simulink model "Follower_V2V_Solyom2013"  (R2014b)
settings: Solver=ode3  SolverMode=SingleTasking  StartTime=0.0  StopTime=10.0  FixedStep=sampleTimes.main  RelTol=1e-3
model workspace (MAT data in the model file):
  spacing = 0
  vehicle = 0
undefined symbols (not defined in the file or in its folder): delays
libraries: simulink x12
settings Model: ParameterArgumentNames=vehicle,spacing  Creator=uos  LastModifiedBy=uos

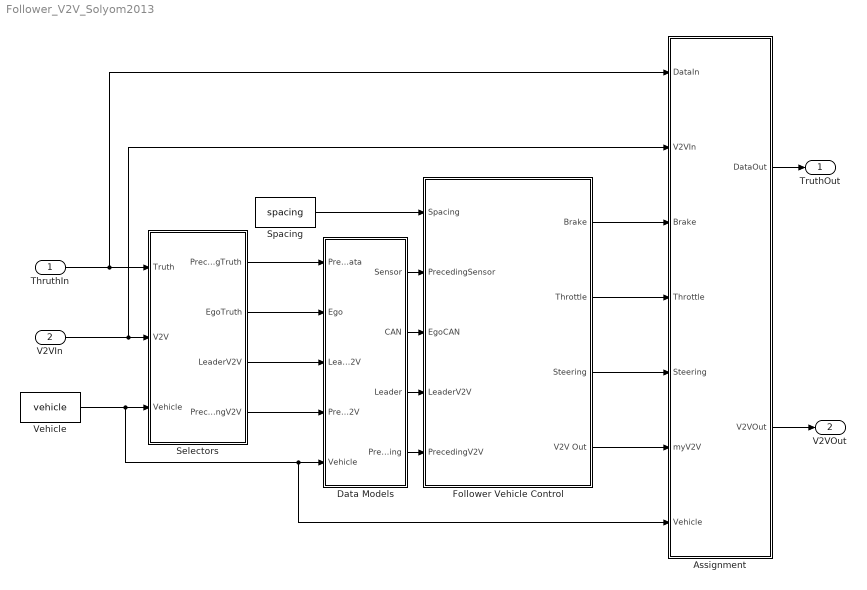
== system Follower_V2V_Solyom2013 ==
  ThruthIn : Inport  OutDataTypeStr=Bus: VehicleBus  PortDimensions=10  BusOutputAsStruct=on
  V2VIn : Inport  Port=2  OutDataTypeStr=Bus: V2VBus  PortDimensions=10  SampleTime=0  BusOutputAsStruct=on
  Assignment : Subsystem
  Data Models : Subsystem
  Follower Vehicle Control : Subsystem
  Selectors : Subsystem
  Spacing : Constant  Value=spacing
  Vehicle : Constant  Value=vehicle
  TruthOut : Outport  OutDataTypeStr=Bus: VehicleBus  PortDimensions=10  BusOutputAsStruct=on
  V2VOut : Outport  Port=2  OutDataTypeStr=Bus: V2VBus  PortDimensions=10  BusOutputAsStruct=on
  wires:
  ThruthIn/1 -> Assignment/1(DataIn), Selectors/1(Truth)
  Assignment/1(DataOut) -> TruthOut/1
  Spacing/1 -> Follower Vehicle Control/1(Spacing)
  Vehicle/1 -> Assignment/7(Vehicle), Data Models/5(Vehicle), Selectors/3(Vehicle)
  Follower Vehicle Control/1(Brake) -> Assignment/3(Brake)
  Follower Vehicle Control/2(Throttle) -> Assignment/4(Throttle)
  Follower Vehicle Control/3(Steering) -> Assignment/5(Steering)
  V2VIn/1 -> Assignment/2(V2VIn), Selectors/2(V2V)
  Assignment/2(V2VOut) -> V2VOut/1
  Follower Vehicle Control/4(V2V Out) -> Assignment/6(myV2V)
  Selectors/1(PrecedingTruth) -> Data Models/1(PrecedingData)
  Selectors/2(EgoTruth) -> Data Models/2(Ego)
  Selectors/3(LeaderV2V) -> Data Models/3(LeaderV2V)
  Selectors/4(PrecedingV2V) -> Data Models/4(PrecedingV2V)
  Data Models/1(Sensor) -> Follower Vehicle Control/2(PrecedingSensor)
  Data Models/2(CAN) -> Follower Vehicle Control/3(EgoCAN)
  Data Models/3(Leader) -> Follower Vehicle Control/4(LeaderV2V)
  Data Models/4(Preceding) -> Follower Vehicle Control/5(PrecedingV2V)

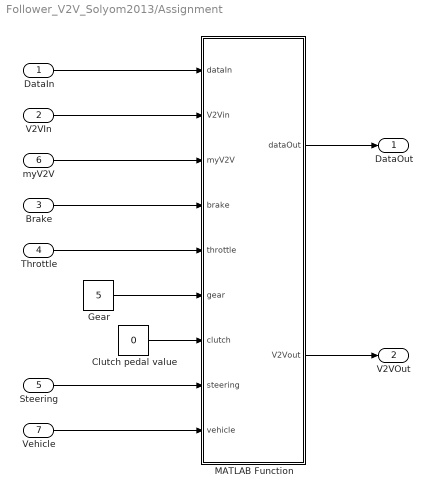
== system Follower_V2V_Solyom2013/Assignment ==
  DataIn : Inport
  V2VIn : Inport  Port=2
  Brake : Inport  Port=3
  Throttle : Inport  Port=4
  Steering : Inport  Port=5
  myV2V : Inport  Port=6
  Vehicle : Inport  Port=7
  Clutch pedal value : Constant  Value=0
  Gear : Constant  Value=5  OutDataTypeStr=int32
  MATLAB Function : MATLAB Function  TreatAsAtomicUnit=on
  DataOut : Outport
  V2VOut : Outport  Port=2
  wires:
  Vehicle/1 -> MATLAB Function/9(vehicle)
  DataIn/1 -> MATLAB Function/1(dataIn)
  Brake/1 -> MATLAB Function/4(brake)
  MATLAB Function/1(dataOut) -> DataOut/1
  Throttle/1 -> MATLAB Function/5(throttle)
  Steering/1 -> MATLAB Function/8(steering)
  V2VIn/1 -> MATLAB Function/2(V2Vin)
  myV2V/1 -> MATLAB Function/3(myV2V)
  MATLAB Function/2(V2Vout) -> V2VOut/1
  Gear/1 -> MATLAB Function/6(gear)
  Clutch pedal value/1 -> MATLAB Function/7(clutch)

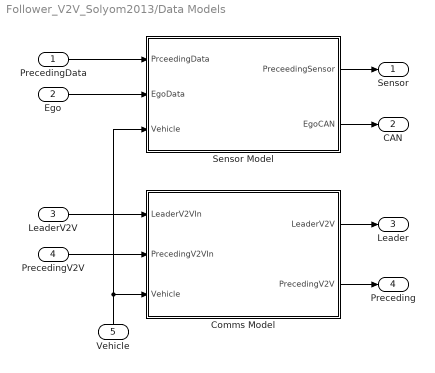
== system Follower_V2V_Solyom2013/Data Models ==
  PrecedingData : Inport
  Ego : Inport  Port=2
  LeaderV2V : Inport  Port=3
  PrecedingV2V : Inport  Port=4
  Vehicle : Inport  Port=5
  Comms Model : Subsystem
  Sensor Model : Subsystem
  Sensor : Outport
  CAN : Outport  Port=2
  Leader : Outport  Port=3
  Preceding : Outport  Port=4
  wires:
  Sensor Model/2(EgoCAN) -> CAN/1
  Sensor Model/1(PreceedingSensor) -> Sensor/1
  PrecedingData/1 -> Sensor Model/1(PrceedingData)
  Ego/1 -> Sensor Model/2(EgoData)
  LeaderV2V/1 -> Comms Model/1(LeaderV2VIn)
  PrecedingV2V/1 -> Comms Model/2(PrecedingV2VIn)
  Comms Model/1(LeaderV2V) -> Leader/1
  Comms Model/2(PrecedingV2V) -> Preceding/1
  Vehicle/1 -> Sensor Model/3(Vehicle), Comms Model/3(Vehicle)

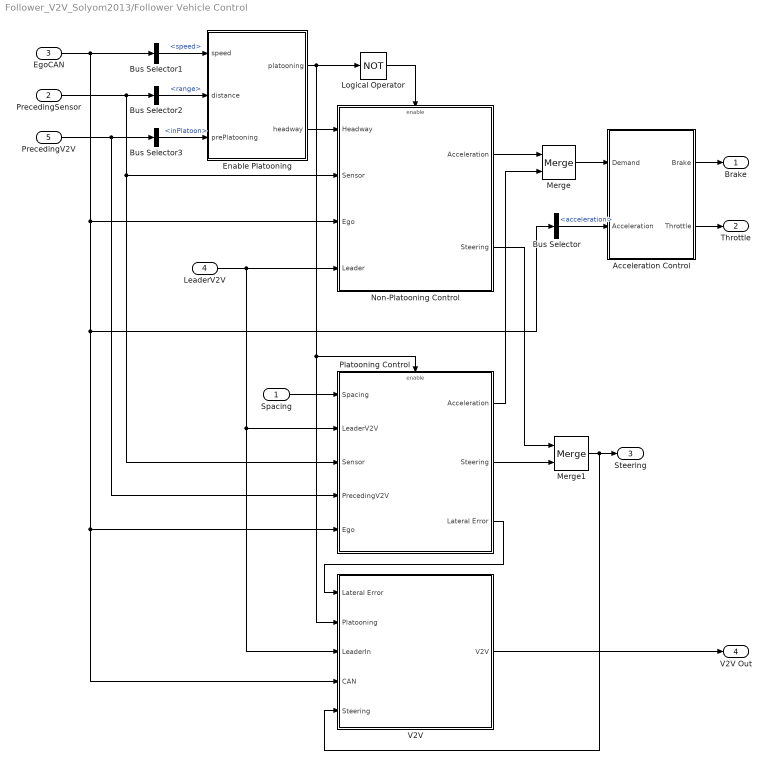
== system Follower_V2V_Solyom2013/Follower Vehicle Control ==
  Spacing : Inport
  PrecedingSensor : Inport  Port=2
  EgoCAN : Inport  Port=3
  LeaderV2V : Inport  Port=4
  PrecedingV2V : Inport  Port=5
  Acceleration Control : Subsystem
  Bus Selector : BusSelector  OutputSignals=acceleration
  Bus Selector1 : BusSelector  OutputSignals=speed
  Bus Selector2 : BusSelector  OutputSignals=range
  Bus Selector3 : BusSelector  OutputSignals=inPlatoon
  Enable Platooning : Stateflow chart  TreatAsAtomicUnit=on
  Logical Operator : Logic  Operator=NOT  AllPortsSameDT=off  OutDataTypeStr=boolean
  Merge : Merge
  Merge1 : Merge
  Non-Platooning Control : Subsystem
  Platooning Control : Subsystem
  V2V : Subsystem
  Brake : Outport
  Throttle : Outport  Port=2
  Steering : Outport  Port=3
  V2V Out : Outport  Port=4
  wires:
  Bus Selector/1 -> Acceleration Control/2(Acceleration)  "<acceleration>"
  Acceleration Control/1(Brake) -> Brake/1
  Acceleration Control/2(Throttle) -> Throttle/1
  Merge1/1 -> Steering/1, V2V/5(Steering)
  Spacing/1 -> Platooning Control/1(Spacing)
  LeaderV2V/1 -> Non-Platooning Control/4(Leader), V2V/3(LeaderIn), Platooning Control/2(LeaderV2V)
  PrecedingSensor/1 -> Platooning Control/3(Sensor), Non-Platooning Control/2(Sensor), Bus Selector2/1
  Merge/1 -> Acceleration Control/1(Demand)
  Platooning Control/1(Acceleration) -> Merge/2
  Non-Platooning Control/1(Acceleration) -> Merge/1
  Platooning Control/2(Steering) -> Merge1/2
  Enable Platooning/1(platooning) -> V2V/2(Platooning), Platooning Control/Enable, Logical Operator/1
  Logical Operator/1 -> Non-Platooning Control/Enable
  Bus Selector1/1 -> Enable Platooning/1(speed)  "<speed>"
  Bus Selector2/1 -> Enable Platooning/2(distance)  "<range>"
  EgoCAN/1 -> Bus Selector1/1, Non-Platooning Control/3(Ego), V2V/4(CAN), Platooning Control/5(Ego), Bus Selector/1
  V2V/1(V2V) -> V2V Out/1
  Enable Platooning/2(headway) -> Non-Platooning Control/1(Headway)
  PrecedingV2V/1 -> Bus Selector3/1, Platooning Control/4(PrecedingV2V)
  Platooning Control/3(Lateral Error) -> V2V/1(Lateral Error)
  Bus Selector3/1 -> Enable Platooning/3(prePlatooning)  "<inPlatoon>"
  Non-Platooning Control/2(Steering) -> Merge1/1

== system Follower_V2V_Solyom2013/Selectors ==
  Truth : Inport
  V2V : Inport  Port=2
  Vehicle : Inport  Port=3
  MATLAB Function : MATLAB Function  TreatAsAtomicUnit=on
  PrecedingTruth : Outport
  EgoTruth : Outport  Port=2
  LeaderV2V : Outport  Port=3
  PrecedingV2V : Outport  Port=4
  wires:
  Truth/1 -> MATLAB Function/1(data)
  Vehicle/1 -> MATLAB Function/3(vehicle)
  MATLAB Function/2(egoTruth) -> EgoTruth/1
  V2V/1 -> MATLAB Function/2(V2V)
  MATLAB Function/3(leaderV2V) -> LeaderV2V/1
  MATLAB Function/4(precedingV2V) -> PrecedingV2V/1
  MATLAB Function/1(precedingTruth) -> PrecedingTruth/1

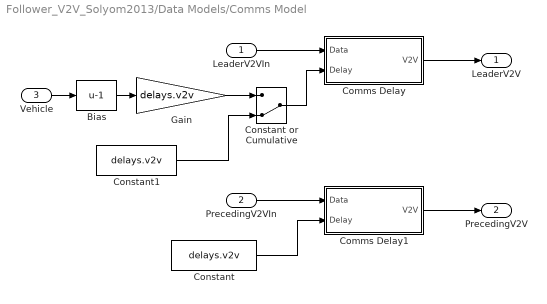
== system Follower_V2V_Solyom2013/Data Models/Comms Model ==
  LeaderV2VIn : Inport
  PrecedingV2VIn : Inport  Port=2
  Vehicle : Inport  Port=3
  Bias : Bias  Bias=-1
  Comms Delay : Subsystem
  Comms Delay1 : Subsystem
  Constant : Constant  Value=delays.v2v
  Constant or Cumulative : ManualSwitch  CurrentSetting=0
  Constant1 : Constant  Value=delays.v2v
  Gain : Gain  Gain=delays.v2v
  LeaderV2V : Outport
  PrecedingV2V : Outport  Port=2
  wires:
  LeaderV2VIn/1 -> Comms Delay/1(Data)
  Comms Delay/1(V2V) -> LeaderV2V/1
  PrecedingV2VIn/1 -> Comms Delay1/1(Data)
  Comms Delay1/1(V2V) -> PrecedingV2V/1
  Constant/1 -> Comms Delay1/2(Delay)
  Constant or Cumulative/1 -> Comms Delay/2(Delay)
  Constant1/1 -> Constant or Cumulative/2
  Vehicle/1 -> Bias/1
  Bias/1 -> Gain/1
  Gain/1 -> Constant or Cumulative/1

== system Follower_V2V_Solyom2013/Data Models/Sensor Model ==
  PrceedingData : Inport
  EgoData : Inport  Port=2
  Vehicle : Inport  Port=3
  CAN Model : Subsystem
  Radar Model : Subsystem
  PreceedingSensor : Outport
  EgoCAN : Outport  Port=2
  wires:
  EgoData/1 -> CAN Model/1(Data), Radar Model/2(Ego)
  Radar Model/1(Radar Data) -> PreceedingSensor/1
  CAN Model/1(CAN) -> EgoCAN/1
  PrceedingData/1 -> Radar Model/1(Target)
  Vehicle/1 -> CAN Model/2(Vehicle)

== system Follower_V2V_Solyom2013/Follower Vehicle Control/Acceleration Control ==
  Demand : Inport
  Acceleration : Inport  Port=2
  Brake Control : Subsystem
  Compare To Constant : simulink/Logic and Bit Operations/Compare To Constant  relop=>=  const=-0.1  OutDataTypeStr=boolean
  Logical Operator : Logic  Operator=NOT  AllPortsSameDT=off  OutDataTypeStr=boolean
  Sum1 : Sum  Inputs=+-|
  Throttle Control : Subsystem
  Brake : Outport
  Throttle : Outport  Port=2
  wires:
  Acceleration/1 -> Throttle Control/2(Acceleration), Sum1/2
  Demand/1 -> Throttle Control/1(Demand), Compare To Constant/1, Sum1/1
  Sum1/1 -> Brake Control/1(Error)
  Brake Control/1(Brake) -> Brake/1
  Throttle Control/1(Throttle) -> Throttle/1
  Compare To Constant/1 -> Throttle Control/Enable, Logical Operator/1
  Logical Operator/1 -> Brake Control/Enable

== system Follower_V2V_Solyom2013/Follower Vehicle Control/Non-Platooning Control ==
  Headway : Inport
  Sensor : Inport  Port=2
  Ego : Inport  Port=3
  Leader : Inport  Port=4
  Enable : EnablePort
  Speed Control : Subsystem
  Steering Control : Subsystem
  Steering Control1 : Subsystem
  Acceleration : Outport
  Steering : Outport  Port=2
  wires:
  Steering Control1/1(Target Curvature) -> Steering Control/2(Target Curvature)
  Ego/1 -> Steering Control/1(Ego), Speed Control/2(Ego)
  Sensor/1 -> Steering Control1/1(Sensor), Speed Control/3(Leader)
  Headway/1 -> Speed Control/1(Headway)
  Speed Control/1(Acceleration Demand) -> Acceleration/1
  Leader/1 -> Steering Control1/2(Leader)
  Steering Control/1(Steering) -> Steering/1

== system Follower_V2V_Solyom2013/Follower Vehicle Control/Platooning Control ==
  Spacing : Inport
  LeaderV2V : Inport  Port=2
  Sensor : Inport  Port=3
  PrecedingV2V : Inport  Port=4
  Ego : Inport  Port=5
  Enable : EnablePort
  Speed Control : Subsystem
  Steering Control : Subsystem
  Acceleration : Outport
  Steering : Outport  Port=2
  Lateral Error : Outport  Port=3
  wires:
  Speed Control/1(Acceleration Demand) -> Acceleration/1
  Spacing/1 -> Speed Control/1(Spacing)
  Sensor/1 -> Steering Control/2(Sensor), Speed Control/3(PreceedingSensor)
  LeaderV2V/1 -> Speed Control/2(LeaderV2V)
  PrecedingV2V/1 -> Steering Control/1(Preceeding), Speed Control/4(PreceedingV2V)
  Ego/1 -> Steering Control/3(Ego), Speed Control/5(Ego)
  Steering Control/1(Steering) -> Steering/1
  Steering Control/2(lateralError1) -> Lateral Error/1

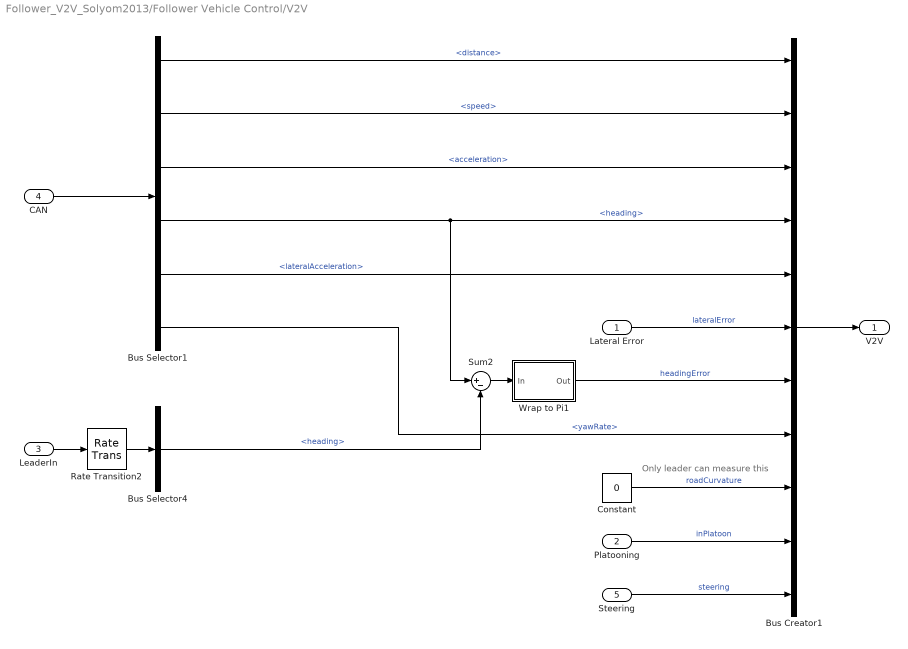
== system Follower_V2V_Solyom2013/Follower Vehicle Control/V2V ==
  note: Only leader can measure this
  Lateral Error : Inport
  Platooning : Inport  Port=2
  LeaderIn : Inport  Port=3
  CAN : Inport  Port=4
  Steering : Inport  Port=5
  Bus Creator1 : BusCreator  Inputs=11  OutDataTypeStr=Bus: V2VBus  NonVirtualBus=on
  Bus Selector1 : BusSelector  OutputSignals=distance,speed,acceleration,heading,lateralAcceleration,yawRate
  Bus Selector4 : BusSelector  OutputSignals=heading
  Constant : Constant  Value=0
  Rate Transition2 : RateTransition  OutPortSampleTime=sampleTimes.control
  Sum2 : Sum  Inputs=|+-
  Wrap to Pi1 : Subsystem
  V2V : Outport
  wires:
  CAN/1 -> Bus Selector1/1
  Bus Selector1/6 -> Bus Creator1/8  "<yawRate>"
  Constant/1 -> Bus Creator1/9  "roadCurvature"
  Bus Selector1/3 -> Bus Creator1/3  "<acceleration>"
  Bus Selector1/1 -> Bus Creator1/1  "<distance>"
  Bus Selector1/2 -> Bus Creator1/2  "<speed>"
  Bus Selector1/5 -> Bus Creator1/5  "<lateralAcceleration>"
  Bus Creator1/1 -> V2V/1
  Bus Selector1/4 -> Bus Creator1/4, Sum2/1  "<heading>"
  Sum2/1 -> Wrap to Pi1/1(In)
  LeaderIn/1 -> Rate Transition2/1
  Rate Transition2/1 -> Bus Selector4/1
  Bus Selector4/1 -> Sum2/2  "<heading>"
  Wrap to Pi1/1(Out) -> Bus Creator1/7  "headingError"
  Lateral Error/1 -> Bus Creator1/6  "lateralError"
  Platooning/1 -> Bus Creator1/10  "inPlatoon"
  Steering/1 -> Bus Creator1/11  "steering"

== system Follower_V2V_Solyom2013/Data Models/Comms Model/Comms Delay ==
  Data : Inport
  Delay : Inport  Port=2
  Display : Display
  Rate Transition1 : RateTransition  OutPortSampleTime=sampleTimes.v2v
  Rate Transition2 : RateTransition  OutPortSampleTime=sampleTimes.main
  Variable Integer Delay : Delay  DelayLengthSource=Input port
      settings: InputPortMap=u0,p1
  Weighted Sample Time Math : SampleTimeMath  TsampMathOp=/
  V2V : Outport
  wires:
  Rate Transition1/1 -> V2V/1
  Data/1 -> Rate Transition2/1
  Rate Transition2/1 -> Variable Integer Delay/1
  Delay/1 -> Weighted Sample Time Math/1
  Weighted Sample Time Math/1 -> Display/1, Variable Integer Delay/2
  Variable Integer Delay/1 -> Rate Transition1/1

== system Follower_V2V_Solyom2013/Data Models/Comms Model/Comms Delay1 ==
  Data : Inport
  Delay : Inport  Port=2
  Rate Transition1 : RateTransition  OutPortSampleTime=sampleTimes.v2v
  Rate Transition2 : RateTransition  OutPortSampleTime=sampleTimes.main
  Variable Integer Delay : Delay  DelayLengthSource=Input port
      settings: InputPortMap=u0,p1
  Weighted Sample Time Math : SampleTimeMath  TsampMathOp=/
  V2V : Outport
  wires:
  Variable Integer Delay/1 -> Rate Transition1/1
  Weighted Sample Time Math/1 -> Variable Integer Delay/2
  Delay/1 -> Weighted Sample Time Math/1
  Rate Transition2/1 -> Variable Integer Delay/1
  Data/1 -> Rate Transition2/1
  Rate Transition1/1 -> V2V/1

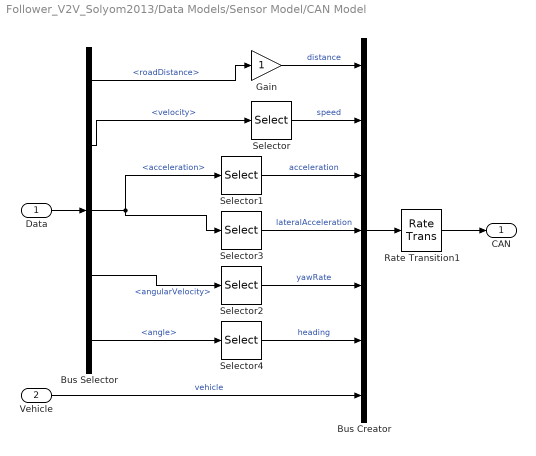
== system Follower_V2V_Solyom2013/Data Models/Sensor Model/CAN Model ==
  Data : Inport
  Vehicle : Inport  Port=2
  Bus Creator : BusCreator  Inputs=7
  Bus Selector : BusSelector  OutputSignals=data.roadDistance,data.velocity,data.acceleration,data.angularVelocity,data.angle
  Gain : Gain
  Rate Transition1 : RateTransition  OutPortSampleTime=sampleTimes.main
  Selector : Selector  InputPortWidth=3
  Selector1 : Selector  InputPortWidth=3
  Selector2 : Selector  InputPortWidth=3  Indices=3
  Selector3 : Selector  InputPortWidth=3  Indices=2
  Selector4 : Selector  InputPortWidth=3  Indices=3
  CAN : Outport
  wires:
  Rate Transition1/1 -> CAN/1
  Bus Creator/1 -> Rate Transition1/1
  Selector1/1 -> Bus Creator/3  "acceleration"
  Bus Selector/3 -> Selector1/1, Selector3/1  "<acceleration>"
  Selector/1 -> Bus Creator/2  "speed"
  Bus Selector/2 -> Selector/1  "<velocity>"
  Data/1 -> Bus Selector/1
  Bus Selector/4 -> Selector2/1  "<angularVelocity>"
  Selector2/1 -> Bus Creator/5  "yawRate"
  Selector3/1 -> Bus Creator/4  "lateralAcceleration"
  Bus Selector/5 -> Selector4/1  "<angle>"
  Selector4/1 -> Bus Creator/6  "heading"
  Bus Selector/1 -> Gain/1  "<roadDistance>"
  Gain/1 -> Bus Creator/1  "distance"
  Vehicle/1 -> Bus Creator/7  "vehicle"

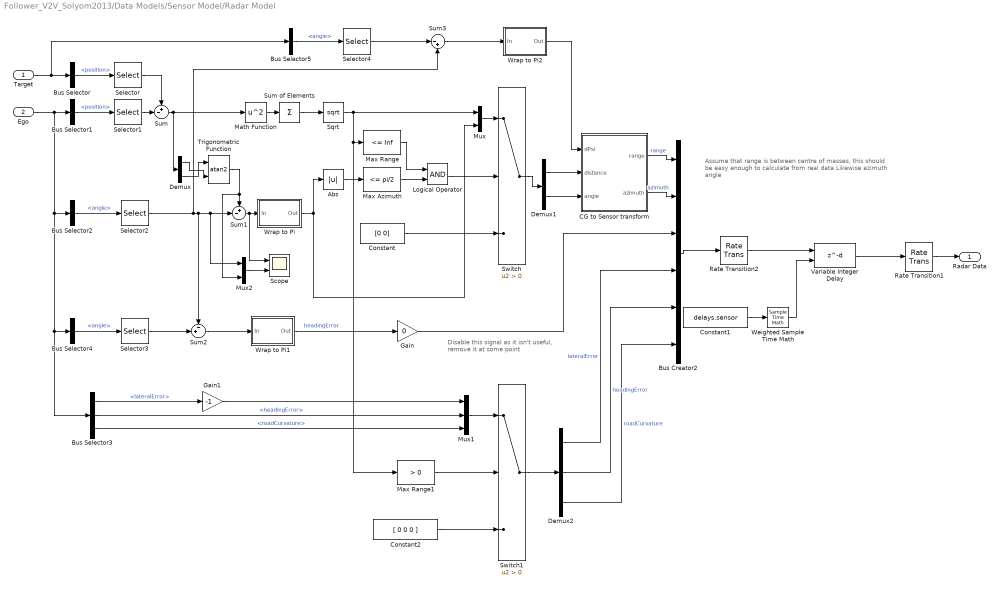
== system Follower_V2V_Solyom2013/Data Models/Sensor Model/Radar Model ==
  note: Assume that range is between centre of masses,
      | this should be easy enough to calculate from real data
      | Likewise azimuth angle
  note: Disable this signal as it isn't useful,
      | remove it at some point
  Target : Inport
  Ego : Inport  Port=2
  Abs : Abs
  Bus Creator2 : BusCreator  Inputs=6
  Bus Selector : BusSelector  OutputSignals=data.position
  Bus Selector1 : BusSelector  OutputSignals=data.position
  Bus Selector2 : BusSelector  OutputSignals=data.angle
  Bus Selector3 : BusSelector  OutputSignals=data.lateralError,data.headingError,data.roadCurvature
  Bus Selector4 : BusSelector  OutputSignals=data.angle
  Bus Selector5 : BusSelector  OutputSignals=data.angle
  CG to Sensor transform : Subsystem
  Constant : Constant  Value=[0 0]
  Constant1 : Constant  Value=delays.sensor
  Constant2 : Constant  Value=[ 0 0 0 ]
  Demux : Demux  Outputs=2
  Demux1 : Demux  Outputs=2
  Demux2 : Demux  Outputs=3
  Gain : Gain  Gain=0
  Gain1 : Gain  Gain=-1
  Logical Operator : Logic  AllPortsSameDT=off  OutDataTypeStr=boolean
  Math Function : Math  Operator=square  SaturateOnIntegerOverflow=on
  Max Azimuth : simulink/Logic and Bit Operations/Compare To Constant  relop=<=  const=pi/2  OutDataTypeStr=boolean
  Max Range : simulink/Logic and Bit Operations/Compare To Constant  relop=<=  const=Inf  OutDataTypeStr=boolean
  Max Range1 : simulink/Logic and Bit Operations/Compare To Constant  relop=>  const=0  OutDataTypeStr=boolean
  Mux : Mux  Inputs=2
  Mux1 : Mux  Inputs=3
  Mux2 : Mux  Inputs=2
  Rate Transition1 : RateTransition  OutPortSampleTime=sampleTimes.sensor
  Rate Transition2 : RateTransition  OutPortSampleTime=sampleTimes.main
  Scope : Scope  NumInputPorts=2
      settings: YMin=-5~-5  YMax=5~5  SaveName=ScopeData11
  Selector : Selector  InputPortWidth=3  Indices=[1 2]
  Selector1 : Selector  InputPortWidth=3  Indices=[1 2]
  Selector2 : Selector  InputPortWidth=3  Indices=3
  Selector3 : Selector  InputPortWidth=3  Indices=3
  Selector4 : Selector  InputPortWidth=3  Indices=3
  Sqrt : Sqrt  SaturateOnIntegerOverflow=on
  Sum : Sum  Inputs=+-|
  Sum of Elements : Sum  Inputs=+
  Sum1 : Sum  Inputs=+-|
  Sum2 : Sum  Inputs=-+|
  Sum3 : Sum  Inputs=|-+
  Switch : Switch  Criteria=u2 > Threshold
  Switch1 : Switch  Criteria=u2 > Threshold
  Trigonometric Function : Trigonometry  Operator=atan2
  Variable Integer Delay : Delay  DelayLengthSource=Input port
      settings: InputPortMap=u0,p1
  Weighted Sample Time Math : SampleTimeMath  TsampMathOp=/
  Wrap to Pi : Subsystem
  Wrap to Pi1 : Subsystem
  Wrap to Pi2 : Subsystem
  Radar Data : Outport
  wires:
  Selector1/1 -> Sum/2
  Selector/1 -> Sum/1
  Bus Selector/1 -> Selector/1  "<position>"
  Bus Selector1/1 -> Selector1/1  "<position>"
  Bus Selector2/1 -> Selector2/1  "<angle>"
  Sum/1 -> Math Function/1, Demux/1
  Selector2/1 -> Sum2/1, Mux2/1, Sum1/2, Sum3/2
  Trigonometric Function/1 -> Mux2/2, Sum1/1
  Sum1/1 -> Scope/1, Wrap to Pi/1(In)
  Math Function/1 -> Sum of Elements/1
  Sum of Elements/1 -> Sqrt/1
  Constant/1 -> Switch/3
  Logical Operator/1 -> Switch/2
  Max Range/1 -> Logical Operator/1
  Abs/1 -> Max Azimuth/1
  Max Azimuth/1 -> Logical Operator/2
  Demux/1 -> Trigonometric Function/2
  Demux/2 -> Trigonometric Function/1
  Wrap to Pi/1(Out) -> Mux/2, Abs/1
  Bus Creator2/1 -> Rate Transition2/1
  Rate Transition1/1 -> Radar Data/1
  Rate Transition2/1 -> Variable Integer Delay/1
  Variable Integer Delay/1 -> Rate Transition1/1
  Constant1/1 -> Weighted Sample Time Math/1
  Weighted Sample Time Math/1 -> Variable Integer Delay/2
  Bus Selector4/1 -> Selector3/1  "<angle>"
  Selector3/1 -> Sum2/2
  Sum2/1 -> Wrap to Pi1/1(In)
  Demux1/2 -> CG to Sensor transform/3(angle)
  Mux/1 -> Switch/1
  Sqrt/1 -> Mux/1, Max Range1/1, Max Range/1
  Switch/1 -> Demux1/1
  Wrap to Pi1/1(Out) -> Gain/1  "headingError"
  Gain/1 -> Bus Creator2/3
  Ego/1 -> Bus Selector2/1, Bus Selector3/1, Bus Selector4/1, Bus Selector1/1
  Mux1/1 -> Switch1/1
  Bus Selector3/1 -> Gain1/1  "<lateralError>"
  Bus Selector3/2 -> Mux1/2  "<headingError>"
  Max Range1/1 -> Switch1/2
  Constant2/1 -> Switch1/3
  Switch1/1 -> Demux2/1
  Demux2/1 -> Bus Creator2/4  "lateralError"
  Demux2/2 -> Bus Creator2/5  "headingError"
  Bus Selector3/3 -> Mux1/3  "<roadCurvature>"
  Demux2/3 -> Bus Creator2/6  "roadCurvature"
  Mux2/1 -> Scope/2
  Gain1/1 -> Mux1/1
  Bus Selector5/1 -> Selector4/1  "<angle>"
  Target/1 -> Bus Selector5/1, Bus Selector/1
  Selector4/1 -> Sum3/1
  Sum3/1 -> Wrap to Pi2/1(In)
  Wrap to Pi2/1(Out) -> CG to Sensor transform/1(dPsi)
  CG to Sensor transform/1(range) -> Bus Creator2/1  "range"
  CG to Sensor transform/2(azimuth) -> Bus Creator2/2  "azimuth"
  Demux1/1 -> CG to Sensor transform/2(distance)

== system Follower_V2V_Solyom2013/Follower Vehicle Control/Acceleration Control/Brake Control ==
  Error : Inport
  Enable : EnablePort  StatesWhenEnabling=reset
  Discrete-Time Integrator : DiscreteIntegrator  InitialConditionSetting=State (most efficient)  SampleTime=-1  LimitOutput=on  UpperSaturationLimit=1  LowerSaturationLimit=-1
  Gain2 : Gain  Gain=0.005
  Gain3 : Gain
  Saturation1 : Saturate  UpperLimit=1  LowerLimit=0
  Sum2 : Sum  Inputs=++|
  Unary Minus : UnaryMinus
  Brake : Outport  OutputWhenDisabled=reset  InitialOutput=0
  wires:
  Saturation1/1 -> Brake/1
  Sum2/1 -> Saturation1/1
  Error/1 -> Unary Minus/1
  Gain2/1 -> Sum2/2
  Discrete-Time Integrator/1 -> Sum2/1
  Gain3/1 -> Discrete-Time Integrator/1
  Unary Minus/1 -> Gain2/1, Gain3/1

== system Follower_V2V_Solyom2013/Follower Vehicle Control/Acceleration Control/Throttle Control ==
  Demand : Inport
  Acceleration : Inport  Port=2
  Enable : EnablePort  StatesWhenEnabling=reset
  Discrete-Time Integrator : DiscreteIntegrator  InitialConditionSetting=State (most efficient)  SampleTime=-1  LimitOutput=on  UpperSaturationLimit=1  LowerSaturationLimit=-1
  Gain : Gain  Gain=1.5
  Gain1 : Gain  Gain=10
  Sum : Sum  Inputs=++|
  Sum1 : Sum  Inputs=+-|
  Throttle : Outport  OutputWhenDisabled=reset  InitialOutput=0
  wires:
  Gain/1 -> Sum/1
  Discrete-Time Integrator/1 -> Sum/2
  Gain1/1 -> Discrete-Time Integrator/1
  Sum/1 -> Throttle/1
  Demand/1 -> Sum1/1, Gain/1
  Acceleration/1 -> Sum1/2
  Sum1/1 -> Gain1/1

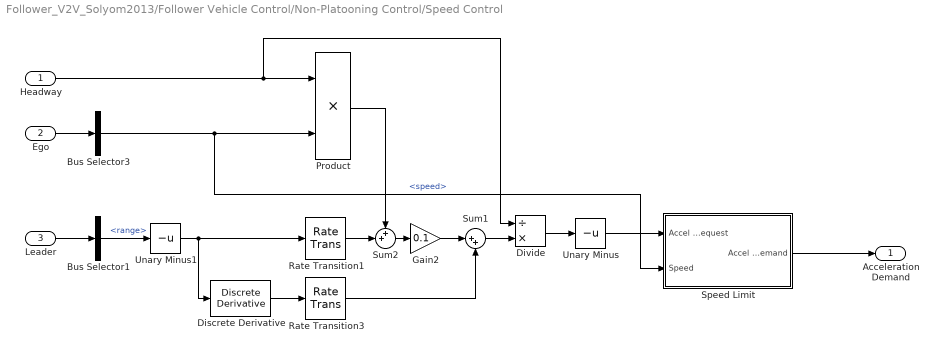
== system Follower_V2V_Solyom2013/Follower Vehicle Control/Non-Platooning Control/Speed Control ==
  Headway : Inport
  Ego : Inport  Port=2
  Leader : Inport  Port=3
  Bus Selector1 : BusSelector  OutputSignals=range
  Bus Selector3 : BusSelector  OutputSignals=speed
  Discrete Derivative : simulink/Discrete/Discrete Derivative  gainval=1.0  ICPrevScaledInput=0.0  InputProcessing=Inherited  OutMin=[]  OutMax=[]  OutDataType=fixdt(1, 16)  OutScaling=2^-10  DoSatur=off
  Divide : Product  Inputs=/*
  Gain2 : Gain  Gain=0.1
  Product : Product
  Rate Transition1 : RateTransition  OutPortSampleTime=sampleTimes.control
  Rate Transition3 : RateTransition  OutPortSampleTime=sampleTimes.control
  Speed Limit : Subsystem
  Sum1 : Sum  Inputs=|++
  Sum2 : Sum  Inputs=++|
  Unary Minus : UnaryMinus
  Unary Minus1 : UnaryMinus
  Acceleration Demand : Outport
  wires:
  Ego/1 -> Bus Selector3/1
  Leader/1 -> Bus Selector1/1
  Bus Selector3/1 -> Speed Limit/2(Speed), Product/2  "<speed>"
  Headway/1 -> Divide/1, Product/1
  Bus Selector1/1 -> Unary Minus1/1  "<range>"
  Product/1 -> Sum2/1
  Sum2/1 -> Gain2/1
  Gain2/1 -> Sum1/1
  Discrete Derivative/1 -> Rate Transition3/1
  Sum1/1 -> Divide/2
  Divide/1 -> Unary Minus/1
  Unary Minus/1 -> Speed Limit/1(Accel Request)
  Rate Transition3/1 -> Sum1/2
  Rate Transition1/1 -> Sum2/2
  Unary Minus1/1 -> Discrete Derivative/1, Rate Transition1/1
  Speed Limit/1(Accel Demand) -> Acceleration Demand/1

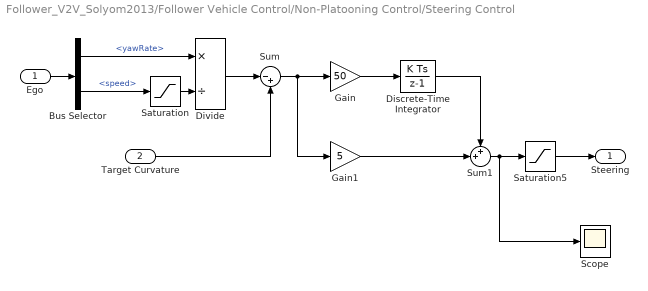
== system Follower_V2V_Solyom2013/Follower Vehicle Control/Non-Platooning Control/Steering Control ==
  Ego : Inport
  Target Curvature : Inport  Port=2
  Bus Selector : BusSelector  OutputSignals=yawRate,speed
  Discrete-Time Integrator : DiscreteIntegrator  InitialCondition=0.0065  InitialConditionSetting=State (most efficient)  SampleTime=-1  LimitOutput=on  UpperSaturationLimit=0.5  LowerSaturationLimit=-0.5
  Divide : Product  Inputs=*/
  Gain : Gain  Gain=50
  Gain1 : Gain  Gain=5
  Saturation : Saturate  UpperLimit=inf  LowerLimit=1
  Saturation5 : Saturate
  Scope : Scope
  Sum : Sum  Inputs=|-+
  Sum1 : Sum  Inputs=++|
  Steering : Outport
  wires:
  Saturation5/1 -> Steering/1
  Sum1/1 -> Scope/1, Saturation5/1
  Target Curvature/1 -> Sum/2
  Ego/1 -> Bus Selector/1
  Bus Selector/2 -> Saturation/1  "<speed>"
  Bus Selector/1 -> Divide/1  "<yawRate>"
  Saturation/1 -> Divide/2
  Divide/1 -> Sum/1
  Gain/1 -> Discrete-Time Integrator/1
  Sum/1 -> Gain/1, Gain1/1
  Gain1/1 -> Sum1/2
  Discrete-Time Integrator/1 -> Sum1/1

== system Follower_V2V_Solyom2013/Follower Vehicle Control/Non-Platooning Control/Steering Control1 ==
  note: Uses the understeer gradient relationship
      | Future work could include learning the gardient as it appears to have a weak dependence on speed
  note: Lateral controller based on curvature
  Sensor : Inport
  Leader : Inport  Port=2
  Add2 : Sum  Inputs=+++
  Bus Selector1 : BusSelector  OutputSignals=headingError,lateralError,roadCurvature
  Bus Selector2 : BusSelector  OutputSignals=lateralError
  Sum : Sum  Inputs=|+-
  kh : Gain  Gain=0.05
  ky : Gain  Gain=0.00075
  Target Curvature : Outport
  wires:
  Sum/1 -> ky/1
  kh/1 -> Add2/1
  ky/1 -> Add2/2
  Add2/1 -> Target Curvature/1
  Sensor/1 -> Bus Selector1/1
  Bus Selector1/1 -> kh/1  "<headingError>"
  Bus Selector1/3 -> Add2/3  "<roadCurvature>"
  Leader/1 -> Bus Selector2/1
  Bus Selector2/1 -> Sum/2  "<lateralError>"
  Bus Selector1/2 -> Sum/1  "<lateralError>"

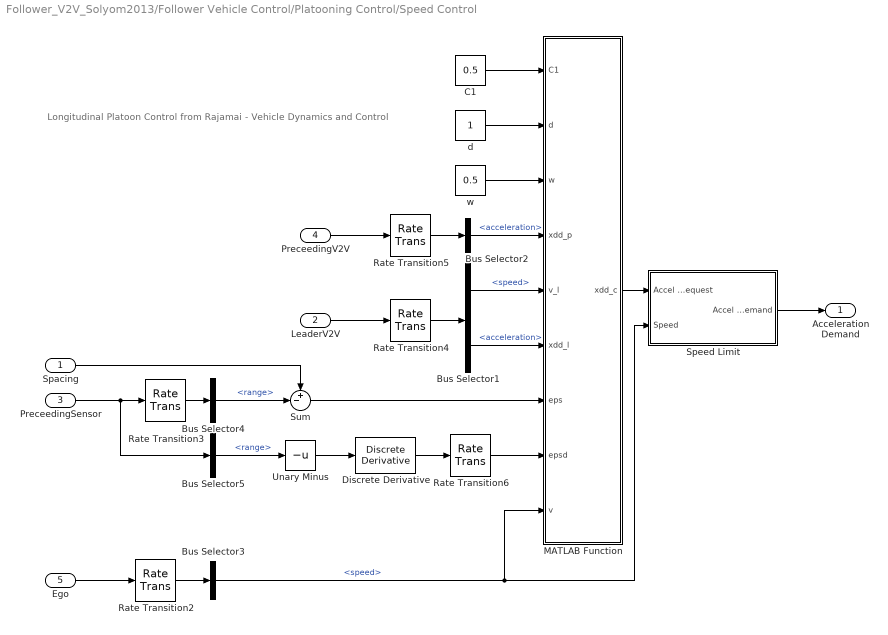
== system Follower_V2V_Solyom2013/Follower Vehicle Control/Platooning Control/Speed Control ==
  note: Longitudinal Platoon Control from Rajamai - Vehicle Dynamics and Control
  Spacing : Inport
  LeaderV2V : Inport  Port=2
  PreceedingSensor : Inport  Port=3
  PreceedingV2V : Inport  Port=4
  Ego : Inport  Port=5
  Bus Selector1 : BusSelector  OutputSignals=speed,acceleration
  Bus Selector2 : BusSelector  OutputSignals=acceleration
  Bus Selector3 : BusSelector  OutputSignals=speed
  Bus Selector4 : BusSelector  OutputSignals=range
  Bus Selector5 : BusSelector  OutputSignals=range
  C1 : Constant  Value=0.5
  Discrete Derivative : simulink/Discrete/Discrete Derivative  gainval=1.0  ICPrevScaledInput=0.0  InputProcessing=Inherited  OutMin=[]  OutMax=[]  OutDataType=fixdt(1, 16)  OutScaling=2^-10  DoSatur=off
  MATLAB Function : MATLAB Function  TreatAsAtomicUnit=on
  Rate Transition2 : RateTransition  OutPortSampleTime=sampleTimes.control
  Rate Transition3 : RateTransition  OutPortSampleTime=sampleTimes.control
  Rate Transition4 : RateTransition  Deterministic=off  OutPortSampleTime=sampleTimes.control
  Rate Transition5 : RateTransition  Deterministic=off  OutPortSampleTime=sampleTimes.control
  Rate Transition6 : RateTransition  Deterministic=off  OutPortSampleTime=sampleTimes.control
  Speed Limit : Subsystem
  Sum : Sum  Inputs=+-|
  Unary Minus : UnaryMinus
  d : Constant
  w : Constant  Value=0.5
  Acceleration Demand : Outport
  wires:
  Ego/1 -> Rate Transition2/1
  Bus Selector3/1 -> Speed Limit/2(Speed), MATLAB Function/9(v)  "<speed>"
  PreceedingSensor/1 -> Bus Selector5/1, Rate Transition3/1
  Bus Selector4/1 -> Sum/2  "<range>"
  Discrete Derivative/1 -> Rate Transition6/1
  Speed Limit/1(Accel Demand) -> Acceleration Demand/1
  C1/1 -> MATLAB Function/1(C1)
  d/1 -> MATLAB Function/2(d)
  w/1 -> MATLAB Function/3(w)
  Spacing/1 -> Sum/1
  LeaderV2V/1 -> Rate Transition4/1
  Bus Selector1/2 -> MATLAB Function/6(xdd_l)  "<acceleration>"
  Bus Selector1/1 -> MATLAB Function/5(v_l)  "<speed>"
  PreceedingV2V/1 -> Rate Transition5/1
  Bus Selector2/1 -> MATLAB Function/4(xdd_p)  "<acceleration>"
  Rate Transition2/1 -> Bus Selector3/1
  Rate Transition3/1 -> Bus Selector4/1
  Rate Transition4/1 -> Bus Selector1/1
  Rate Transition5/1 -> Bus Selector2/1
  Bus Selector5/1 -> Unary Minus/1  "<range>"
  Rate Transition6/1 -> MATLAB Function/8(epsd)
  Sum/1 -> MATLAB Function/7(eps)
  Unary Minus/1 -> Discrete Derivative/1
  MATLAB Function/1(xdd_c) -> Speed Limit/1(Accel Request)

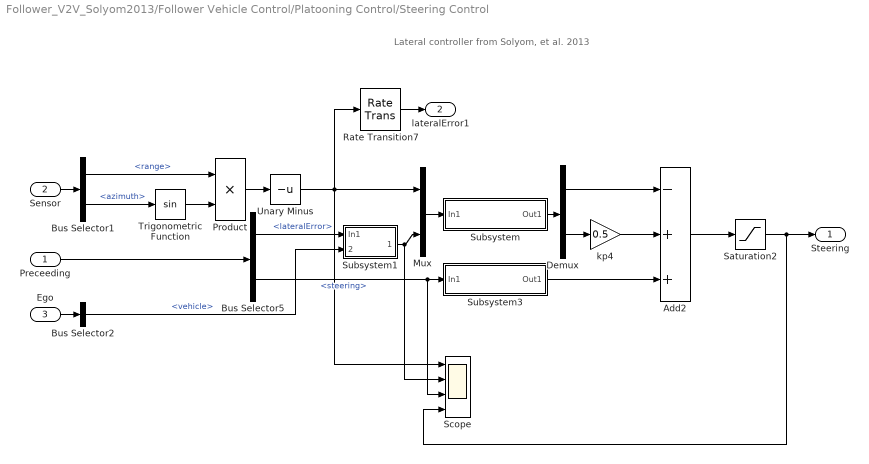
== system Follower_V2V_Solyom2013/Follower Vehicle Control/Platooning Control/Steering Control ==
  note: Lateral controller from Solyom, et al. 2013
  Preceeding : Inport
  Sensor : Inport  Port=2
  Ego : Inport  Port=3
  Add2 : Sum  Inputs=-++
  Bus Selector1 : BusSelector  OutputSignals=range,azimuth
  Bus Selector2 : BusSelector  OutputSignals=vehicle
  Bus Selector5 : BusSelector  OutputSignals=lateralError,steering
  Demux : Demux  Outputs=2
  Mux : Mux  Inputs=2
  Product : Product
  Rate Transition7 : RateTransition  Integrity=off  Deterministic=off  OutPortSampleTime=sampleTimes.control
  Saturation2 : Saturate
  Scope : Scope  NumInputPorts=4
      settings: TimeRange=30  YMin=5.9975~-0.0015~-0.2~-5  YMax=6.001~0.001~0.6~5  SaveName=Errors
  Subsystem : Subsystem
  Subsystem1 : Subsystem
  Subsystem3 : Subsystem
  Trigonometric Function : Trigonometry
  Unary Minus : UnaryMinus
  kp4 : Gain  Gain=0.5
  Steering : Outport
  lateralError1 : Outport  Port=2
  wires:
  kp4/1 -> Add2/2
  Subsystem/1(Out1) -> Demux/1
  Demux/1 -> Add2/1
  Product/1 -> Unary Minus/1
  Mux/1 -> Subsystem/1(In1)
  Subsystem3/1(Out1) -> Add2/3
  Sensor/1 -> Bus Selector1/1
  Bus Selector1/1 -> Product/1  "<range>"
  Bus Selector5/2 -> Scope/3, Subsystem3/1(In1)  "<steering>"
  Bus Selector5/1 -> Subsystem1/1(In1)  "<lateralError>"
  Saturation2/1 -> Scope/4, Steering/1
  Demux/2 -> kp4/1
  Add2/1 -> Saturation2/1
  Preceeding/1 -> Bus Selector5/1
  Bus Selector1/2 -> Trigonometric Function/1  "<azimuth>"
  Trigonometric Function/1 -> Product/2
  Rate Transition7/1 -> lateralError1/1
  Unary Minus/1 -> Rate Transition7/1, Scope/1, Mux/1
  Subsystem1/1(Out1) -> Mux/2, Scope/2
  Ego/1 -> Bus Selector2/1
  Bus Selector2/1 -> Subsystem1/2(Vehicle)  "<vehicle>"

== system Follower_V2V_Solyom2013/Follower Vehicle Control/V2V/Wrap to Pi1 ==
  In : Inport
  Bias : Bias  Bias=pi
  Bias1 : Bias  Bias=-pi
  Constant : Constant  Value=2*pi
  Math Function : Math  Operator=mod  SaturateOnIntegerOverflow=on
  Out : Outport
  wires:
  Constant/1 -> Math Function/2
  Bias1/1 -> Out/1
  Math Function/1 -> Bias1/1
  Bias/1 -> Math Function/1
  In/1 -> Bias/1

== system Follower_V2V_Solyom2013/Data Models/Sensor Model/Radar Model/CG to Sensor transform ==
  dPsi : Inport
  distance : Inport  Port=2
  angle : Inport  Port=3
  MATLAB Function : MATLAB Function  TreatAsAtomicUnit=on
  range : Outport
  azimuth : Outport  Port=2
  wires:
  distance/1 -> MATLAB Function/1(d)
  angle/1 -> MATLAB Function/2(theta)
  dPsi/1 -> MATLAB Function/3(dpsi)
  MATLAB Function/1(d_r) -> range/1
  MATLAB Function/2(theta_c) -> azimuth/1

== system Follower_V2V_Solyom2013/Data Models/Sensor Model/Radar Model/Wrap to Pi ==
  In : Inport
  Bias : Bias  Bias=pi
  Bias1 : Bias  Bias=-pi
  Constant : Constant  Value=2*pi
  Math Function : Math  Operator=mod  SaturateOnIntegerOverflow=on
  Out : Outport
  wires:
  In/1 -> Bias/1
  Bias/1 -> Math Function/1
  Math Function/1 -> Bias1/1
  Bias1/1 -> Out/1
  Constant/1 -> Math Function/2

== system Follower_V2V_Solyom2013/Data Models/Sensor Model/Radar Model/Wrap to Pi1 ==
  In : Inport
  Bias : Bias  Bias=pi
  Bias1 : Bias  Bias=-pi
  Constant : Constant  Value=2*pi
  Math Function : Math  Operator=mod  SaturateOnIntegerOverflow=on
  Out : Outport
  wires:
  Constant/1 -> Math Function/2
  Bias1/1 -> Out/1
  Math Function/1 -> Bias1/1
  Bias/1 -> Math Function/1
  In/1 -> Bias/1

== system Follower_V2V_Solyom2013/Data Models/Sensor Model/Radar Model/Wrap to Pi2 ==
  In : Inport
  Bias : Bias  Bias=pi
  Bias1 : Bias  Bias=-pi
  Constant : Constant  Value=2*pi
  Math Function : Math  Operator=mod  SaturateOnIntegerOverflow=on
  Out : Outport
  wires:
  Constant/1 -> Math Function/2
  Bias1/1 -> Out/1
  Math Function/1 -> Bias1/1
  Bias/1 -> Math Function/1
  In/1 -> Bias/1

== system Follower_V2V_Solyom2013/Follower Vehicle Control/Non-Platooning Control/Speed Control/Speed Limit ==
  Accel Request : Inport
  Speed : Inport  Port=2
  70mph : simulink/Logic and Bit Operations/Compare To Constant  relop=<  const=31.3  OutDataTypeStr=boolean
  Compare To Zero : simulink/Logic and Bit Operations/Compare To Zero  relop=<  OutDataTypeStr=boolean
  Constant3 : Constant  Value=0
  Logical Operator : Logic  Operator=OR  AllPortsSameDT=off  OutDataTypeStr=boolean
  Switch : Switch  Criteria=u2 > Threshold
  Accel Demand : Outport
  wires:
  Speed/1 -> 70mph/1
  Compare To Zero/1 -> Logical Operator/1
  Logical Operator/1 -> Switch/2
  70mph/1 -> Logical Operator/2
  Constant3/1 -> Switch/3
  Accel Request/1 -> Compare To Zero/1, Switch/1
  Switch/1 -> Accel Demand/1

== system Follower_V2V_Solyom2013/Follower Vehicle Control/Platooning Control/Speed Control/Speed Limit ==
  Accel Request : Inport
  Speed : Inport  Port=2
  70mph : simulink/Logic and Bit Operations/Compare To Constant  relop=<  const=31.3  OutDataTypeStr=boolean
  Compare To Zero : simulink/Logic and Bit Operations/Compare To Zero  relop=<  OutDataTypeStr=boolean
  Constant3 : Constant  Value=0
  Logical Operator : Logic  Operator=OR  AllPortsSameDT=off  OutDataTypeStr=boolean
  Switch : Switch  Criteria=u2 > Threshold
  Accel Demand : Outport
  wires:
  Speed/1 -> 70mph/1
  Compare To Zero/1 -> Logical Operator/1
  Logical Operator/1 -> Switch/2
  70mph/1 -> Logical Operator/2
  Constant3/1 -> Switch/3
  Accel Request/1 -> Compare To Zero/1, Switch/1
  Switch/1 -> Accel Demand/1

== system Follower_V2V_Solyom2013/Follower Vehicle Control/Platooning Control/Steering Control/Subsystem ==
  In1 : Inport
  Discrete Derivative : simulink/Discrete/Discrete Derivative  gainval=1.0  ICPrevScaledInput=0.0  InputProcessing=Inherited  OutMin=[]  OutMax=[]  OutDataType=fixdt(1, 16)  OutScaling=2^-10  DoSatur=off
  Gain : Gain  Gain=0.2
  Gain1 : Gain  Gain=0.01
  Sum : Sum  Inputs=|++
  Out1 : Outport
  wires:
  In1/1 -> Gain/1, Gain1/1
  Sum/1 -> Out1/1
  Gain1/1 -> Discrete Derivative/1
  Discrete Derivative/1 -> Sum/2
  Gain/1 -> Sum/1

== system Follower_V2V_Solyom2013/Follower Vehicle Control/Platooning Control/Steering Control/Subsystem1 ==
  In1 : Inport
  Vehicle : Inport  Port=2
  Compare To Constant : simulink/Logic and Bit Operations/Compare To Constant  relop=>=  const=3.0  OutDataTypeStr=boolean
  Constant : Constant  Value=0
  Switch : Switch  Criteria=u2 > Threshold
  Out1 : Outport
  wires:
  In1/1 -> Switch/1
  Switch/1 -> Out1/1
  Vehicle/1 -> Compare To Constant/1
  Compare To Constant/1 -> Switch/2
  Constant/1 -> Switch/3

== system Follower_V2V_Solyom2013/Follower Vehicle Control/Platooning Control/Steering Control/Subsystem3 ==
  In1 : Inport
  Discrete Transfer Fcn : DiscreteTransferFcn  Numerator="[-0.0531    0.1961   -0.1834    0.0558   -0.0001]"  Denominator="[1.0000   -2.6653    2.7034   -1.2409    0.2180]"
  Out1 : Outport
  wires:
  Discrete Transfer Fcn/1 -> Out1/1
  In1/1 -> Discrete Transfer Fcn/1

== matlab function Follower_V2V_Solyom2013/Assignment/MATLAB Function ==
  data: dataIn input Bus: VehicleBus size=10; V2Vin input Bus: V2VBus size=10; myV2V input Bus: V2VBus size=1; brake input size=1; throttle input; gear input; clutch input; steering input; dataOut output Bus: VehicleBus size=10; vehicle input; V2Vout output Bus: V2VBus size=10
function [dataOut, V2Vout]  = fcn(dataIn, V2Vin, myV2V, brake,throttle,gear,clutch,steering, vehicle)
%#codegen

dataOut = dataIn;
dataOut(vehicle).control.brake = brake;
dataOut(vehicle).control.throttle = throttle;
dataOut(vehicle).control.clutch = clutch;
dataOut(vehicle).control.steering = steering;
dataOut(vehicle).control.gear = gear;

V2Vout = V2Vin;
V2Vout(vehicle) = myV2V;

== matlab function Follower_V2V_Solyom2013/Selectors/MATLAB Function ==
  data: precedingTruth output Bus: VehicleBus size=1; egoTruth output Bus: VehicleBus size=1; leaderV2V output Bus: V2VBus size=1; data input Bus: VehicleBus size=10; V2V input Bus: V2VBus size=10; precedingV2V output Bus: V2VBus size=1; vehicle input
function [precedingTruth, egoTruth, leaderV2V, precedingV2V] = fcn(data, V2V, vehicle)
%#codegen

if (vehicle > 1)
    precedingTruth = data(vehicle-1);
    precedingV2V = V2V(vehicle-1);
else
    error('There is no preceeding vehicle!');
end
egoTruth = data(vehicle);

leaderV2V = V2V(1);

== stateflow chart Follower_V2V_Solyom2013/Follower Vehicle Control/Enable Platooning ==
  state NotPlatooning
    en: platooning = logical(0);
    state GainSpeed
      en: headway = 1;
    state CloseDistance
      en: headway = 0.5;
    (default) -> GainSpeed
    GainSpeed -> CloseDistance : after(30,sec)[speed>10]
  state Platooning
    en: platooning = logical(1);
  (default) -> NotPlatooning
  CloseDistance -> Platooning : [prePlatooning && distance < 15]
  data: platooning output boolean; speed input; distance input; headway output; prePlatooning input boolean

== matlab function Follower_V2V_Solyom2013/Data Models/Sensor Model/Radar Model/CG to Sensor transform/MATLAB Function ==
  data: d input; d_r output; theta input; dpsi input; theta_c output
function [d_r, theta_c] = fcn(d,theta,dpsi)
%#codegen

lb = 2.5;
lr = 1;
lc = 1;


A = d*sin(theta)/sin(dpsi);
B = d*sin(dpsi-theta)/sin(dpsi);

d_r = sqrt((A-lb)^2 + (B-lr)^2 + 2*(A-lb)*(B-lr)*cos(dpsi));

d_c = sqrt((A-lb)^2 + (B-lc)^2 + 2*(A-lb)*(B-lc)*cos(dpsi));

theta_c = asin(sin(dpsi)*(A-lb)/d_c);

== matlab function Follower_V2V_Solyom2013/Follower Vehicle Control/Platooning Control/Speed Control/MATLAB Function ==
  data: C1 input; d input; w input; xdd_p input; v_l input; xdd_c output; xdd_l input; eps input; epsd input; v input
function xdd_c = fcn(C1, d, w, xdd_p, v_l, xdd_l, eps, epsd, v)
%#codegen

% From Rajamani - Vehicle Dynamics and Control

xdd_c = (1-C1)*xdd_p + C1*xdd_l - (2*d - C1*(d + sqrt(d*d - 1)))*w*epsd ...
    - (d + sqrt(d*d - 1))*w*C1*(v-v_l) - w*w*eps;
